simulink model "case1_simu"  (R2015a)
settings: Solver=ode45  StartTime=0.0  StopTime=10  RelTol=1e-3
settings Model: Creator=jesus  LastModifiedBy=jesus

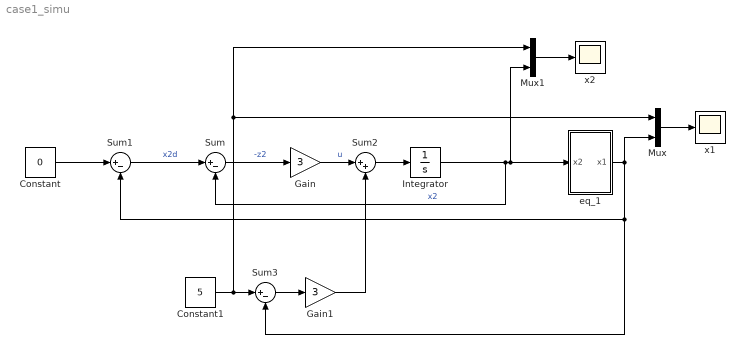
== system case1_simu ==
  Constant : Constant  Value=0
  Constant1 : Constant  Value=5
  Gain : Gain  Gain=3
  Gain1 : Gain  Gain=3
  Integrator : Integrator  InitialCondition=1
  Mux : Mux  Inputs=2
  Mux1 : Mux  Inputs=2
  Sum : Sum  Inputs=|+-
  Sum1 : Sum  Inputs=|+-
  Sum2 : Sum  Inputs=|++
  Sum3 : Sum  Inputs=|+-
  eq_1 : Subsystem
  x1 : Scope
  x2 : Scope
  wires:
  Integrator/1 -> Sum/2, Mux1/2, eq_1/1(x2)  "x2"
  Sum/1 -> Gain/1  "-z2"
  Sum1/1 -> Sum/1  "x2d"
  eq_1/1(x1) -> Sum1/2, Sum3/2, Mux/2
  Constant/1 -> Sum1/1
  Mux/1 -> x1/1
  Mux1/1 -> x2/1
  Gain/1 -> Sum2/1  "u"
  Sum2/1 -> Integrator/1
  Sum3/1 -> Gain1/1
  Gain1/1 -> Sum2/2
  Constant1/1 -> Mux1/1, Mux/1, Sum3/1

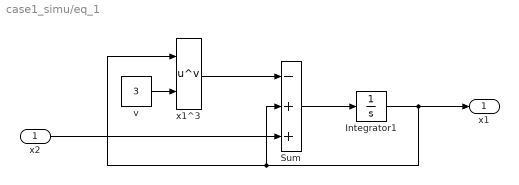
== system case1_simu/eq_1 ==
  x2 : Inport
  Integrator1 : Integrator  InitialCondition=1
  Sum : Sum  Inputs=-++
  v : Constant  Value=3
  x1^3 : Math  Operator=pow  SaturateOnIntegerOverflow=on
  x1 : Outport
  wires:
  Sum/1 -> Integrator1/1
  v/1 -> x1^3/2
  x1^3/1 -> Sum/1
  Integrator1/1 -> x1/1, x1^3/1, Sum/2
  x2/1 -> Sum/3
